simulink model "rstanu"  (R2013a)
settings: Solver=ode45  StartTime=0.0  StopTime=10.0  RelTol=1e-3
values from neighbouring files (symbols this model uses):
  cp = 1000    [skrypt.m]
  Cv1 = cp*gp*V1    (= 90000)    [skrypt.m]
  Cv2 = cp*gp*V2    (= 144000)    [skrypt.m]
  czas_skoku = 300    [skrypt.m]
  dTkz = 0    [skrypt.m]
  dTzew = 0    [skrypt.m]
  fk = fkN*0.5    (= 0.194444444444)    [skrypt.m]
  gp = 1.2    [skrypt.m]
  K0 = (cp*gp*fkN*0.7*(TkzN - T1N)) / (T1N - T2N)    (= 653.333333333)    [skrypt.m]
  K1 = (cp*gp*fkN*0.3*(TkzN-T1N)) / (T1N - TzewN)    (= 35)    [skrypt.m]
  K2 = ((cp*gp*fkN + K0)*(T1N-T2N)) / (T2N - TzewN)    (= 160)    [skrypt.m]
  T10 = (cp*gp*fk*Tkz + K1*Tzew + ((K0*K2*Tzew)/(K0+K2+cp*gp*fk))) / (cp*gp*fk + K1 + K0 - ((K0*(K0+cp*gp*fk))/(K0+K2+cp*gp*fk)))    [skrypt.m]
  T20 = ((K0+cp*gp*fk)*T10 + K2*Tzew) / (K0 + cp*gp*fk + K2)    [skrypt.m]
  Tkz = TkzN    (= 30)    [skrypt.m]
  Tzew = TzewN+i*5    [skrypt.m]
settings Model: Creator=LAB320-1552  LastModifiedBy=LAB320-1552

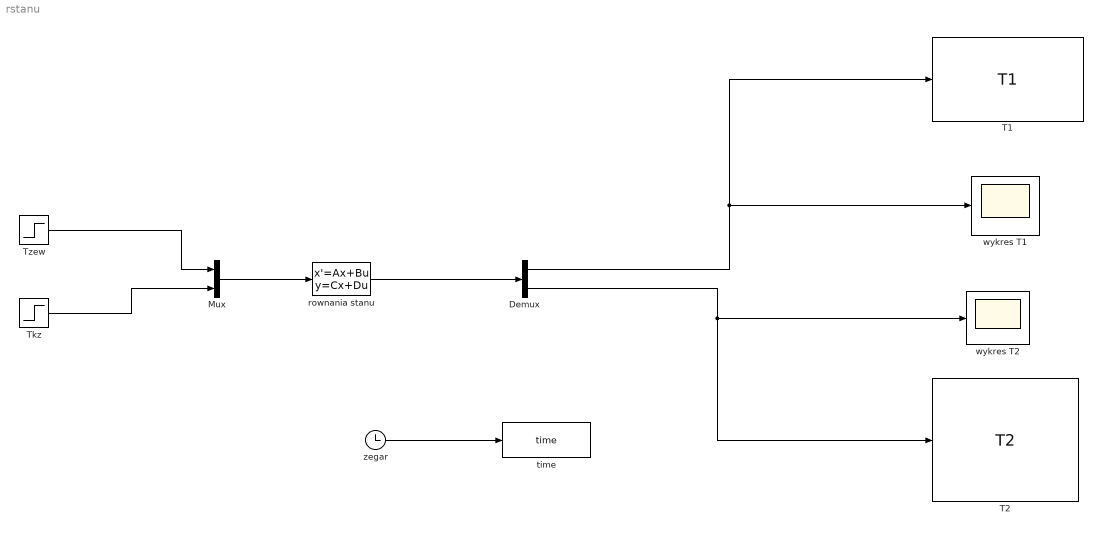
== system rstanu ==
  Demux : Demux  Outputs=2
  Mux : Mux  Inputs=2
  T1 : ToWorkspace  VariableName=T1  SampleTime=-1
  T2 : ToWorkspace  VariableName=T2  SampleTime=-1
  Tkz : Step  Time=czas_skoku  Before=Tkz  After=Tkz+dTkz  SampleTime=0
  Tzew : Step  Time=czas_skoku  Before=Tzew  After=Tzew+dTzew  SampleTime=0
  rownania stanu : StateSpace  A=[(-(cp*gp*fk+K1+K0)/Cv1) (K0/Cv1); ((K0+cp*gp*fk)/Cv2) (-(K0+cp*gp*fk+K2)/Cv2)]  B=[K1/Cv1 cp*gp*fk/Cv1; K2/Cv2 0]  C=[1 0; 0 1]  D=[0 0;0 0]  X0=[T10; T20]
  time : ToWorkspace  VariableName=time  SampleTime=-1
  wykres T1 : Scope
  wykres T2 : Scope
  zegar : Clock
  wires:
  rownania stanu/1 -> Demux/1
  Demux/1 -> T1/1, wykres T1/1
  Demux/2 -> T2/1, wykres T2/1
  zegar/1 -> time/1
  Mux/1 -> rownania stanu/1
  Tkz/1 -> Mux/2
  Tzew/1 -> Mux/1
